simulink model "model"  (R2017a)
settings: Solver=ode45  StartTime=0.0  StopTime=4  RelTol=1e-3  EnableMultiTasking=on
libraries: simulink x1
settings Model: Creator=Javier  LastModifiedBy=javier
settings DataIOCC: LimitDataPoints=on  SaveFormat=Array
settings OptimizationCC: LifeSpan=inf
settings DebuggingCC: SolverPrmCheckMsg=warning  SFUnexpectedBacktrackingDiag=warning  SFNoUnconditionalDefaultTransitionDiag=warning  SFExecutionAtInitializationDiag=none
settings HardwareCC: ProdBitPerPointer=32  ProdBitPerSizeT=32  ProdBitPerPtrDiffT=32  ProdLargestAtomicFloat=None  ProdIntDivRoundTo=Undefined  ProdEndianess=Unspecified  ProdWordSize=32  ProdHWDeviceType=32-bit Generic
settings ModelReferenceCC: PropagateSignalLabelsOutOfModel=off
settings GRTTargetCC: TargetLangStandard=C89/C90 (ANSI)  GeneratePreprocessorConditionals=Disable all
settings ConfigComp: CovMetricSettings=dw  CovHtmlReporting=on  CovSaveCumulativeToWorkspaceVar=on  CovSaveSingleToWorkspaceVar=on  CovExternalEMLEnable=off  CovSFcnEnable=off

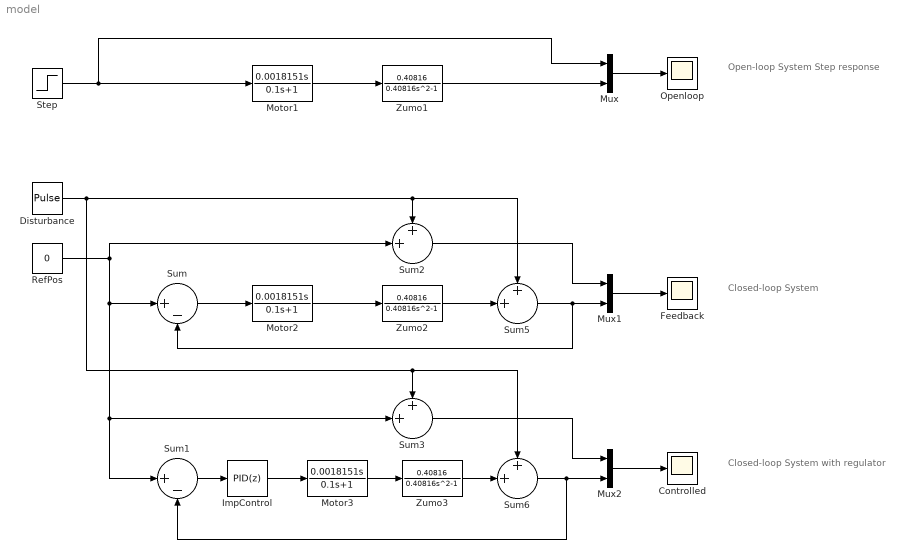
== system model ==
  note: Open-loop System
      | Step response
  note: Closed-loop System
  note: Closed-loop System with regulator
  Controlled : Scope
  Disturbance : DiscretePulseGenerator  PulseType=Time based  Amplitude=0.1  Period=5  PulseWidth=0.01  PhaseDelay=0.2
  Feedback : Scope
  ImpControl : simulink/Continuous/PID Controller  Controller=PID  TimeDomain=Discrete-time  SampleTime=-1  IntegratorMethod=Forward Euler  FilterMethod=Forward Euler  Form=Parallel  UseFilter=off  ControllerParametersSource=internal  P=1  I=1  D=0  N=170.253284410686  InitialConditionSource=internal  InitialConditionForIntegrator=0  InitialConditionForFilter=0  ExternalReset=none  LimitOutput=off  UpperSaturationLimit=inf  LowerSaturationLimit=-inf  LinearizeAsGain=on  AntiWindupMode=none  Kb=1  TrackingMode=off  Kt=1  PParamMin=[]  PParamMax=[]  IParamMin=[]  IParamMax=[]  DParamMin=[]  DParamMax=[]  NParamMin=[]  NParamMax=[]  KbParamMin=[]  KbParamMax=[]  KtParamMin=[]  KtParamMax=[]  POutMin=[]  POutMax=[]  IOutMin=[]  IOutMax=[]  DOutMin=[]  DOutMax=[]  NOutMin=[]  NOutMax=[]  KbOutMin=[]  KbOutMax=[]  KtOutMin=[]  KtOutMax=[]  IntegratorOutMin=[]  IntegratorOutMax=[]  FilterOutMin=[]  FilterOutMax=[]  SumOutMin=[]  SumOutMax=[]  SumI1OutMin=[]  SumI1OutMax=[]  SumI2OutMin=[]  SumI2OutMax=[]  SumI3OutMin=[]  SumI3OutMax=[]  SumDOutMin=[]  SumDOutMax=[]  SaturationOutMin=[]  SaturationOutMax=[]  IntegratorContinuousStateAttributes=''  IntegratorStateMustResolveToSignalObject=off  IntegratorRTWStateStorageClass=Auto  FilterContinuousStateAttributes=''  FilterStateMustResolveToSignalObject=off  FilterRTWStateStorageClass=Auto  DifferentiatorICPrevScaledInput=0  DifferentiatorOutMin=[]  DifferentiatorOutMax=[]  InitialConditionSetting=State (most efficient)
  Motor1 : TransferFcn  Numerator=[0.0018151 0]  Denominator=[0.1 1]
  Motor2 : TransferFcn  Numerator=[0.0018151 0]  Denominator=[0.1 1]
  Motor3 : TransferFcn  Numerator=[0.0018151 0]  Denominator=[0.1 1]
  Mux : Mux  Inputs=2
  Mux1 : Mux  Inputs=2
  Mux2 : Mux  Inputs=2
  Openloop : Scope
  RefPos : Constant  Value=0
  Step : Step  Time=0.2  After=5  SampleTime=0
  Sum : Sum  Inputs=|+-
  Sum1 : Sum  Inputs=|+-
  Sum{2..3,5..6} (4 alike) : Sum  Inputs=++|
  Zumo1 : TransferFcn  Numerator=0.40816  Denominator=[0.40816 0 -1]
  Zumo2 : TransferFcn  Numerator=0.40816  Denominator=[0.40816 0 -1]
  Zumo3 : TransferFcn  Numerator=0.40816  Denominator=[0.40816 0 -1]
  wires:
  Motor1/1 -> Zumo1/1
  RefPos/1 -> Sum1/1, Sum3/2, Sum/1, Sum2/2
  Sum/1 -> Motor2/1
  Motor2/1 -> Zumo2/1
  Mux1/1 -> Feedback/1
  Mux/1 -> Openloop/1
  Motor3/1 -> Zumo3/1
  ImpControl/1 -> Motor3/1
  Sum1/1 -> ImpControl/1
  Mux2/1 -> Controlled/1
  Disturbance/1 -> Sum3/1, Sum6/1, Sum2/1, Sum5/1
  Zumo2/1 -> Sum5/2
  Sum5/1 -> Sum/2, Mux1/2
  Zumo3/1 -> Sum6/2
  Sum6/1 -> Sum1/2, Mux2/2
  Step/1 -> Mux/1, Motor1/1
  Sum2/1 -> Mux1/1
  Sum3/1 -> Mux2/1
  Zumo1/1 -> Mux/2
